simulink model "sim_env"  (R2023b)
settings: Solver=VariableStepAuto  StartTime=0.0  StopTime=10  RelTol=1e-3
values from neighbouring files (symbols this model uses):
  cg_z = 0.335    [para_sim1dot4.mat]    (also in para_sim1dot5.mat; para_sim1dot6.mat = 0.215; para_sim1dot7.mat = 0.215)
  F35thrust = [0 0.011 0.018 0.024 0.031 0.037 0.046 0.053 0.061 0.07 0.079 0.088 ... (170 elements, 85x2)]    [para_sim1dot3.mat]    (also in para_sim1dot4.mat; para_sim1dot5.mat; para_sim1dot6.mat; para_sim1dot7.mat)
  fin_drag_over_v2 = [-30 -25 -20 -15 -10 -5 0 5 10 15 20 25 ... (26 elements, 13x2)]    [para_sim1dot2.mat]    (also in para_sim1dot3.mat; para_sim1dot4.mat; para_sim1dot5.mat; para_sim1dot6.mat)
  fin_lift_over_v2 = [-30 -25 -20 -15 -10 -5 0 5 10 15 20 25 ... (26 elements, 13x2)]    [para_sim1dot2.mat]    (also in para_sim1dot3.mat; para_sim1dot4.mat; para_sim1dot5.mat; para_sim1dot6.mat)
  l_arm_moment = 0.5    [para_sim1dot2.mat]    (also in para_sim1dot3.mat; para_sim1dot4.mat = 0.3; para_sim1dot5.mat = 0.3; para_sim1dot6.mat = 0.175)
  mass = 1    [para_sim1dot0.mat]    (also in para_sim1dot1.mat; para_sim1dot2.mat = 0.6; para_sim1dot3.mat = 0.8; para_sim1dot4.mat = 0.8)
  r_arm_moment = 0.05    [para_sim1dot2.mat]    (also in para_sim1dot3.mat; para_sim1dot4.mat; para_sim1dot5.mat; para_sim1dot6.mat = 0.065)
libraries: simulink_extras x7, simulink x3, shared6dof x1, aerolibanim x1, matrix_library x1, aerolibanimutils x1
settings Model: Creator=Zian Liu  LastModifiedBy=Zian Liu

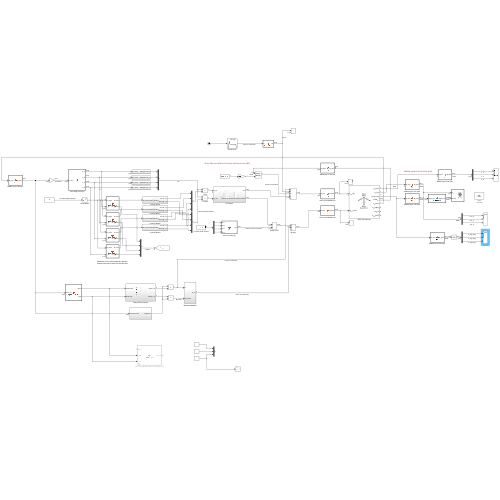
[thumbnail: Simulink's stored preview of the top-level diagram]
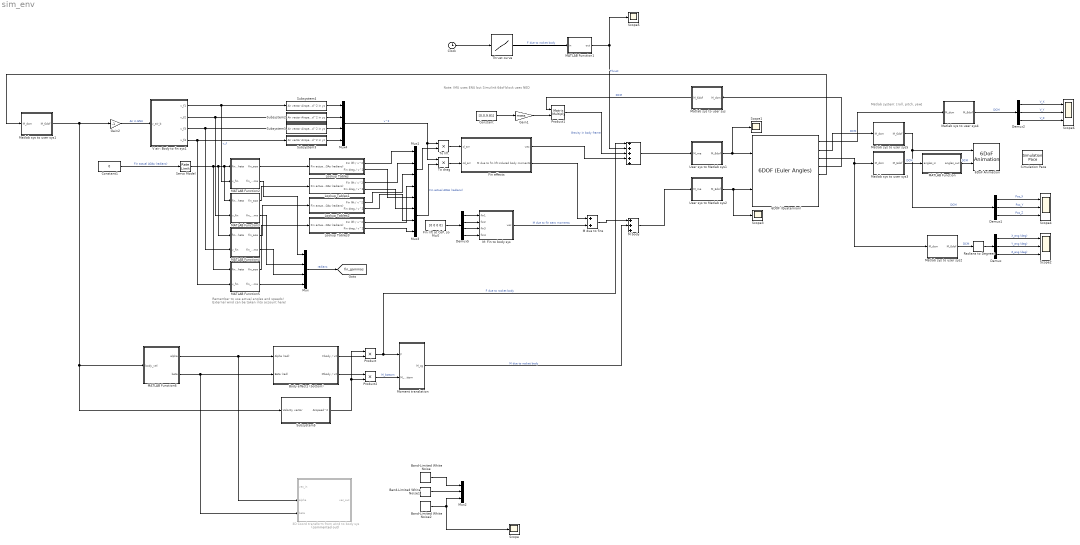
== system sim_env ==
  note: Matlab system: [roll, pitch, yaw]
  note: Note: IMU uses ENU but Simulink 6dof block uses NED
  note: Remember to use actual angles and speeds!
      | External wind can be taken into account here!
  " " : Sum  Inputs=+++++
  3D Coord transform from wind to body sys : MATLAB Function  Commented=on  TreatAsAtomicUnit=on
  6DOF (Quaternion) : shared6dof/6DOF (Euler Angles)  units=Metric (MKS)  mtype=Fixed  rep=Quaternion  xme_0=[0 0 0]  Vm_0=[0 0 0]  eul_0=[0 0 0]  pm_0=[0 0 0]  mass_0=mass  mass_e=0.5  mass_f=2.0  inertia=diag([0.0301315, 0.0301315, 0.0004096])  inertia_e=eye(3)  inertia_f=2*eye(3)  k_quat=1.0  vre_flag=on  abi_flag=off  aMode=0  xme_statename=''  Vm_statename=''  eul_statename=''  quat_statename={'qr', 'qi', 'qj','qk'}  pm_statename=''  mass_statename=''
      settings: LibrarySourceBlock=aerolib6dof2/6DOF (Quaternion)
  6DoF Animation : aerolibanim/6DoF Animation  u1=[-100 100 -100 100 -300 300]  u2=0.1  u3=100  u4=[10000 0 0]  u5=Fly alongside  u6=[10000 0 0]  u7=0  u8=off
  Band-Limited White Noise : simulink/Sources/Band-Limited White Noise  Cov=[0.1]  Ts=0.01  seed=[23341]
  Band-Limited White Noise1 : simulink/Sources/Band-Limited White Noise  Cov=[0.1]  Ts=0.01  seed=[23342]
  Band-Limited White Noise2 : simulink/Sources/Band-Limited White Noise  Cov=[0.1]  Ts=0.01  seed=[23343]
  Body effects (bottom) : Subsystem
  Clock : Clock
  Constant : Constant  Value=[0,0,9.81]
  Constant1 : Constant  Value=0
  Demux : Demux  Outputs=3
  Demux1 : Demux  Outputs=3
  Demux2 : Demux  Outputs=3
  Demux5 : Demux
  Fin effects : Subsystem
  "Fin lift at CoP, so M=0" : Constant  Value=[0 0 0 0]
  Gain1 : Gain  Gain=mass
  Gain2 : Gain  Gain=-1
  Lookup Tables : Subsystem
  Lookup Tables1 : Subsystem
  Lookup Tables2 : Subsystem
  Lookup Tables3 : Subsystem
  M body : Sum  Inputs=+++
  M due to fins : Sum
  M: Fin to body sys : MATLAB Function  TreatAsAtomicUnit=on
  MATLAB Function : MATLAB Function  TreatAsAtomicUnit=on
  MATLAB Function1 : MATLAB Function  TreatAsAtomicUnit=on
  MATLAB Function2 : MATLAB Function  TreatAsAtomicUnit=on
  MATLAB Function3 : MATLAB Function  TreatAsAtomicUnit=on
  MATLAB Function4 : MATLAB Function  TreatAsAtomicUnit=on
  MATLAB Function5 : MATLAB Function  TreatAsAtomicUnit=on
  MATLAB Function6 : MATLAB Function  TreatAsAtomicUnit=on
  Matlab sys to user sys : MATLAB Function  TreatAsAtomicUnit=on
  Matlab sys to user sys1 : MATLAB Function  TreatAsAtomicUnit=on
  Matlab sys to user sys2 : MATLAB Function  TreatAsAtomicUnit=on
  Matlab sys to user sys3 : MATLAB Function  TreatAsAtomicUnit=on
  Matlab sys to user sys4 : MATLAB Function  TreatAsAtomicUnit=on
  Matlab sys to user sys5 : MATLAB Function  TreatAsAtomicUnit=on
  Moment translation : Subsystem
  Mux{,1,3..4} (4 alike) : Mux
  Mux2 : Mux  Inputs=3
  Product : Product
  Product1 : Product  Multiplication=Matrix(*)
  Product2 : Product
  Radians to Degrees : simulink_extras/Transformations/Radians to Degrees
  Scope{,1,3,5} (4 alike) : Scope
  Scope2 : Scope  NumInputPorts=3
  Scope4 : Scope  NumInputPorts=3
  Scope6 : Scope  NumInputPorts=3
  Servo Model : RateLimiter  SampleTimeMode=inherited
  Simulation Pace : aerolibanimutils/Simulation Pace  SimulationPace=1  SleepMode=Auto  OutputPaceError=off  SampleTime=1/30
  Subsystem1 : Subsystem
  Subsystem2 : Subsystem
  Subsystem3 : Subsystem
  Subsystem4 : Subsystem
  Subsystem5 : Subsystem
  Thrust curve : Lookup_n-D  NumberOfTableDimensions=1  BreakpointsForDimension1=F35thrust(:,1)  Table=F35thrust(:,2)  ExtrapMethod=Clip  InternalRulePriority=Speed  RndMeth=Simplest
  To drag : Product
  To lift : Product
  User sys to Matlab sys1 : MATLAB Function  TreatAsAtomicUnit=on
  User sys to Matlab sys2 : MATLAB Function  TreatAsAtomicUnit=on
  V air: Body to fin sys1 : MATLAB Function  TreatAsAtomicUnit=on
  tag scope: fin_gammas=global
  wires:
  Matlab sys to user sys1/1(M_6dof) -> Subsystem5/1(Velocity vector), MATLAB Function6/1(body_vel), Gain2/1
  Gain2/1 -> V air: Body to fin sys1/1(v_air_b)  "Air in ENU"
  Subsystem1/1(Airspeed^2 in yz) -> Mux4/3
  Subsystem2/1(Airspeed^2 in yz) -> Mux4/2
  Mux1/1 -> To lift/2
  V air: Body to fin sys1/4(v_f4) -> Subsystem3/1(Air vector), MATLAB Function5/2(v_fin)
  Subsystem4/1(Airspeed^2 in yz) -> Mux4/1
  Matlab sys to user sys/1(M_6dof) -> Product1/1  "DCM"
  Constant1/1 -> Servo Model/1  "Fin actual AOAs (radians)"
  6DOF (Quaternion)/3 -> Matlab sys to user sys2/1(M_dcm), Matlab sys to user sys3/1(M_dcm)
  Subsystem3/1(Airspeed^2 in yz) -> Mux4/4
  Gain1/1 -> Product1/2
  M due to fins/1 -> M body/1
  " "/1 -> User sys to Matlab sys1/1(M_me)
  User sys to Matlab sys2/1(M_6dof) -> Scope3/1, 6DOF (Quaternion)/2
  Constant/1 -> Gain1/1
  "Fin lift at CoP, so M=0"/1 -> Demux5/1
  M body/1 -> User sys to Matlab sys2/1(M_me)
  V air: Body to fin sys1/3(v_f3) -> Subsystem1/1(Air vector), MATLAB Function4/2(v_fin)
  Moment translation/1(M_cg) -> M body/2  "M due to rocket body"
  Demux5/2 -> M: Fin to body sys/2(fin2)
  Demux5/3 -> M: Fin to body sys/3(fin3)
  Thrust curve/1 -> MATLAB Function1/1(in)  "F due to rocket body"
  Demux5/1 -> M: Fin to body sys/1(fin1)
  Demux5/4 -> M: Fin to body sys/4(fin4)
  M: Fin to body sys/1(vec) -> M due to fins/2  "M due to fin aero moments"
  User sys to Matlab sys1/1(M_6dof) -> 6DOF (Quaternion)/1, Scope1/1
  Mux4/1 -> To drag/1, To lift/1  "v^2"
  Product1/1 -> " "/3  "Gravity in body frame"
  6DOF (Quaternion)/4 -> Matlab sys to user sys/1(M_dcm)
  6DOF (Quaternion)/5 -> Matlab sys to user sys1/1(M_dcm)
  Matlab sys to user sys2/1(M_6dof) -> Radians to Degrees/1  "DCM"
  6DOF (Quaternion)/2 -> Matlab sys to user sys5/1(M_dcm)  "DCM"
  Clock/1 -> Thrust curve/1
  MATLAB Function1/1(out) -> Scope5/1, " "/2  "Thrust"
  MATLAB Function/1(angles_out) -> 6DoF Animation/2  "DCM"
  Matlab sys to user sys3/1(M_6dof) -> MATLAB Function/1(angles_in)  "DCM"
  Matlab sys to user sys5/1(M_6dof) -> Demux1/1, 6DoF Animation/1  "DCM"
  V air: Body to fin sys1/1(v_f1) -> Subsystem4/1(Air vector), MATLAB Function2/2(v_fin)  "v_f"
  V air: Body to fin sys1/2(v_f2) -> Subsystem2/1(Air vector), MATLAB Function3/2(v_fin)
  Demux/3 -> Scope2/3  "Z_ang (deg)"
  Demux/2 -> Scope2/2  "Y_ang (deg)"
  Demux/1 -> Scope2/1  "X_ang (deg)"
  Demux1/3 -> Scope4/3  "Pos_Z"
  Demux1/1 -> Scope4/1  "Pos_X"
  Demux1/2 -> Scope4/2  "Pos_Y"
  MATLAB Function2/1(fin_aoa) -> Lookup Tables/1(Fin actual AOAs (radians))
  MATLAB Function3/1(fin_aoa) -> Lookup Tables1/1(Fin actual AOAs (radians))
  MATLAB Function4/1(fin_aoa) -> Lookup Tables2/1(Fin actual AOAs (radians))
  MATLAB Function5/1(fin_aoa) -> Lookup Tables3/1(Fin actual AOAs (radians))
  MATLAB Function6/1(alpha) -> 3D Coord transform from wind to body sys/2(alpha), Body effects (bottom)/1(Alpha (rad))
  MATLAB Function6/2(beta) -> 3D Coord transform from wind to body sys/3(beta), Body effects (bottom)/2(Beta (rad))
  MATLAB Function5/2(fin_gamma) -> Mux/4
  To lift/1 -> Fin effects/1(cl_arr)
  To drag/1 -> Fin effects/2(cd_arr)
  Fin effects/1(vec) -> " "/4
  Fin effects/2(M due to fin lift induced body moments) -> M due to fins/1
  Mux/1 -> [fin_gammas]  "radians"
  MATLAB Function4/2(fin_gamma) -> Mux/3
  MATLAB Function3/2(fin_gamma) -> Mux/2
  MATLAB Function2/2(fin_gamma) -> Mux/1
  Band-Limited White Noise/1 -> Mux2/1
  Band-Limited White Noise2/1 -> Scope/1, Mux2/3
  Band-Limited White Noise1/1 -> Mux2/2
  Demux2/3 -> Scope6/3  "V_Z"
  Demux2/2 -> Scope6/2  "V_Y"
  Demux2/1 -> Scope6/1  "V_X"
  6DOF (Quaternion)/1 -> Matlab sys to user sys4/1(M_dcm)
  Matlab sys to user sys4/1(M_6dof) -> Demux2/1  "DCM"
  Servo Model/1 -> MATLAB Function5/1(fin_theta), MATLAB Function4/1(fin_theta), MATLAB Function3/1(fin_theta), MATLAB Function2/1(fin_theta)
  Lookup Tables/1(Fin lift / v^2) -> Mux1/1
  Lookup Tables1/1(Fin lift / v^2) -> Mux1/2
  Lookup Tables2/1(Fin lift / v^2) -> Mux1/3
  Lookup Tables3/1(Fin lift / v^2) -> Mux1/4
  Lookup Tables/2(Fin drag / v^2) -> Mux3/1
  Lookup Tables1/2(Fin drag / v^2) -> Mux3/2
  Lookup Tables2/2(Fin drag / v^2) -> Mux3/3
  Lookup Tables3/2(Fin drag / v^2) -> Mux3/4
  Mux3/1 -> To drag/2  "Fin actual AOAs (radians)"
  Radians to Degrees/1 -> Demux/1
  Product2/1 -> Moment translation/2(M_bottom)  "M_bottom"
  Product/1 -> Moment translation/1(F), " "/1  "F due to rocket body"
  Body effects (bottom)/1(Fbody / v2) -> Product/2
  Body effects (bottom)/2(Mbody / v2) -> Product2/1
  Subsystem5/1(Airspeed^2) -> Product/1, Product2/2

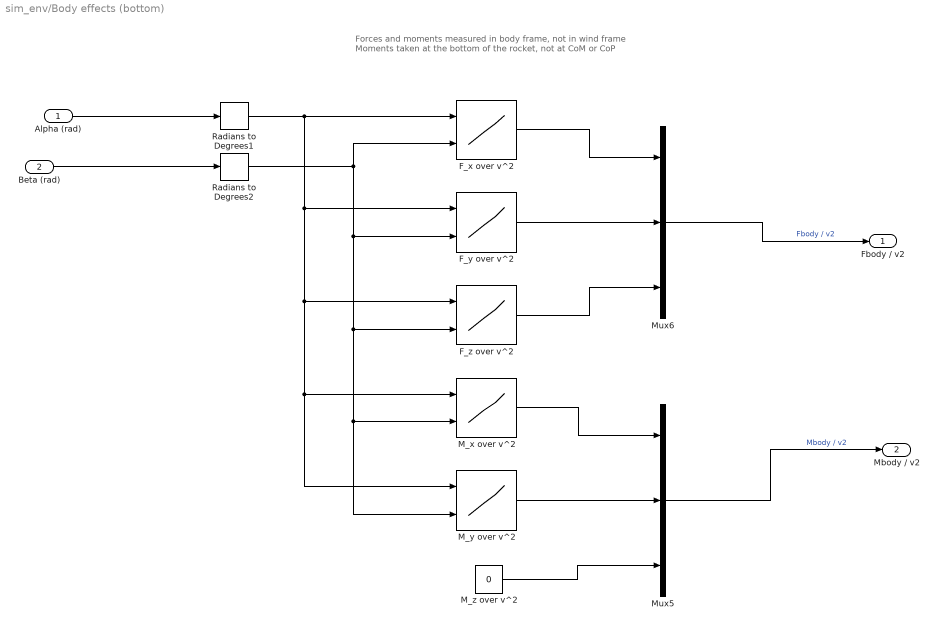
== system sim_env/Body effects (bottom) ==
  note: Forces and moments measured in body frame, not in wind frame
      |
      | Moments taken at the bottom of the rocket, not at CoM or CoP
  Alpha (rad) : Inport
  Beta (rad) : Inport  Port=2
  F_x over v^2 : Lookup_n-D  BreakpointsForDimension1=body_Fx_over_v2(2:end,1)  BreakpointsForDimension2=body_Fx_over_v2(1,2:end)  BreakpointsForDimension3=[5, 7]  Table=body_Fx_over_v2(2:end,2:end)  ExtrapMethod=Clip  InternalRulePriority=Speed  RndMeth=Simplest
      settings: InputPortMap=u0,u1
  F_y over v^2 : Lookup_n-D  BreakpointsForDimension1=body_Fy_over_v2(2:end,1)  BreakpointsForDimension2=body_Fy_over_v2(1,2:end)  BreakpointsForDimension3=[5, 7]  Table=body_Fy_over_v2(2:end,2:end)  ExtrapMethod=Clip  InternalRulePriority=Speed  RndMeth=Simplest
      settings: InputPortMap=u0,u1
  F_z over v^2 : Lookup_n-D  BreakpointsForDimension1=body_Fz_over_v2(2:end,1)  BreakpointsForDimension2=body_Fz_over_v2(1,2:end)  BreakpointsForDimension3=[5, 7]  Table=body_Fz_over_v2(2:end,2:end)  ExtrapMethod=Clip  InternalRulePriority=Speed  RndMeth=Simplest
      settings: InputPortMap=u0,u1
  M_x over v^2 : Lookup_n-D  BreakpointsForDimension1=body_Mx_over_v2(2:end,1)  BreakpointsForDimension2=body_Mx_over_v2(1,2:end)  BreakpointsForDimension3=[5, 7]  Table=body_Mx_over_v2(2:end,2:end)  ExtrapMethod=Clip  InternalRulePriority=Speed  RndMeth=Simplest
      settings: InputPortMap=u0,u1
  M_y over v^2 : Lookup_n-D  BreakpointsForDimension1=body_My_over_v2(2:end,1)  BreakpointsForDimension2=body_My_over_v2(1,2:end)  BreakpointsForDimension3=[5, 7]  Table=body_My_over_v2(2:end,2:end)  ExtrapMethod=Clip  InternalRulePriority=Speed  RndMeth=Simplest
      settings: InputPortMap=u0,u1
  M_z over v^2 : Constant  Value=0
  Mux5 : Mux  Inputs=3
  Mux6 : Mux  Inputs=3
  Radians to Degrees1 : simulink_extras/Transformations/Radians to Degrees
  Radians to Degrees2 : simulink_extras/Transformations/Radians to Degrees
  Fbody / v2 : Outport
  Mbody / v2 : Outport  Port=2
  wires:
  F_y over v^2/1 -> Mux6/2
  M_x over v^2/1 -> Mux5/1
  Radians to Degrees1/1 -> M_y over v^2/1, M_x over v^2/1, F_z over v^2/1, F_y over v^2/1, F_x over v^2/1
  Radians to Degrees2/1 -> F_x over v^2/2, M_y over v^2/2, M_x over v^2/2, F_z over v^2/2, F_y over v^2/2
  F_x over v^2/1 -> Mux6/1
  Mux6/1 -> Fbody / v2/1  "Fbody / v2"
  M_y over v^2/1 -> Mux5/2
  Alpha (rad)/1 -> Radians to Degrees1/1
  M_z over v^2/1 -> Mux5/3
  F_z over v^2/1 -> Mux6/3
  Mux5/1 -> Mbody / v2/1  "Mbody / v2"
  Beta (rad)/1 -> Radians to Degrees2/1

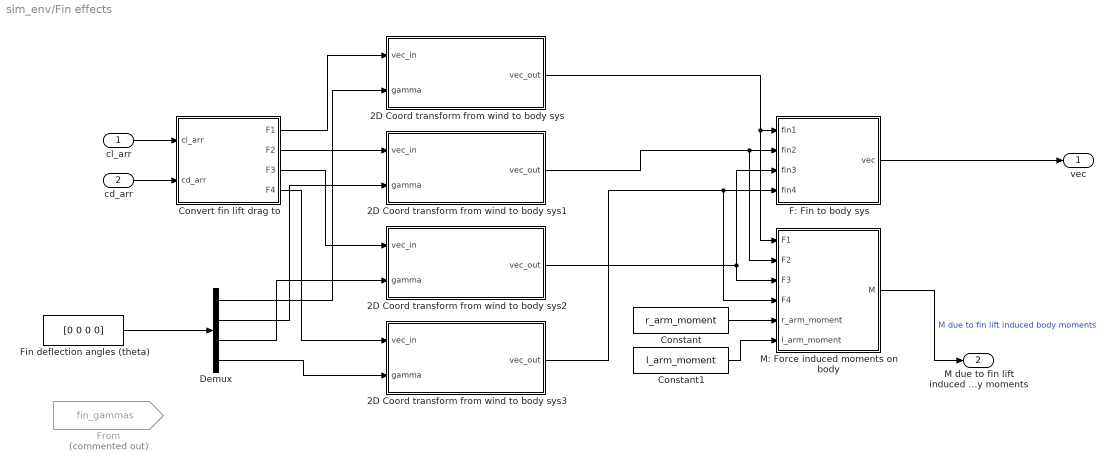
== system sim_env/Fin effects ==
  cl_arr : Inport
  cd_arr : Inport  Port=2
  2D Coord transform from wind to body sys : MATLAB Function  TreatAsAtomicUnit=on
  2D Coord transform from wind to body sys1 : MATLAB Function  TreatAsAtomicUnit=on
  2D Coord transform from wind to body sys2 : MATLAB Function  TreatAsAtomicUnit=on
  2D Coord transform from wind to body sys3 : MATLAB Function  TreatAsAtomicUnit=on
  Constant : Constant  Value=r_arm_moment
  Constant1 : Constant  Value=l_arm_moment
  "Convert fin lift drag to " : MATLAB Function  TreatAsAtomicUnit=on
  Demux : Demux
  F: Fin to body sys : MATLAB Function  TreatAsAtomicUnit=on
  Fin deflection angles (theta) : Constant  Value=[0 0 0 0]
  From : From  Commented=on  GotoTag=fin_gammas  TagVisibility=global
  M: Force induced moments on body : MATLAB Function  TreatAsAtomicUnit=on
  vec : Outport
  M due to fin lift induced body moments : Outport  Port=2
  wires:
  2D Coord transform from wind to body sys/1(vec_out) -> M: Force induced moments on body/1(F1), F: Fin to body sys/1(fin1)
  2D Coord transform from wind to body sys2/1(vec_out) -> F: Fin to body sys/3(fin3), M: Force induced moments on body/3(F3)
  2D Coord transform from wind to body sys3/1(vec_out) -> M: Force induced moments on body/4(F4), F: Fin to body sys/4(fin4)
  cl_arr/1 -> "Convert fin lift drag to "/1(cl_arr)
  2D Coord transform from wind to body sys1/1(vec_out) -> M: Force induced moments on body/2(F2), F: Fin to body sys/2(fin2)
  F: Fin to body sys/1(vec) -> vec/1
  M: Force induced moments on body/1(M) -> M due to fin lift induced body moments/1  "M due to fin lift induced body moments"
  cd_arr/1 -> "Convert fin lift drag to "/2(cd_arr)
  "Convert fin lift drag to "/1(F1) -> 2D Coord transform from wind to body sys/1(vec_in)
  "Convert fin lift drag to "/2(F2) -> 2D Coord transform from wind to body sys1/1(vec_in)
  "Convert fin lift drag to "/3(F3) -> 2D Coord transform from wind to body sys2/1(vec_in)
  "Convert fin lift drag to "/4(F4) -> 2D Coord transform from wind to body sys3/1(vec_in)
  Fin deflection angles (theta)/1 -> Demux/1
  Demux/4 -> 2D Coord transform from wind to body sys3/2(gamma)
  Demux/3 -> 2D Coord transform from wind to body sys2/2(gamma)
  Demux/2 -> 2D Coord transform from wind to body sys1/2(gamma)
  Demux/1 -> 2D Coord transform from wind to body sys/2(gamma)
  Constant/1 -> M: Force induced moments on body/5(r_arm_moment)
  Constant1/1 -> M: Force induced moments on body/6(l_arm_moment)

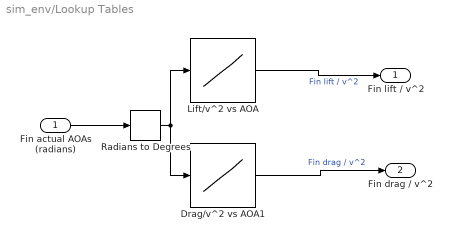
== system sim_env/Lookup Tables ==
  Fin actual AOAs (radians) : Inport
  Drag/v^2 vs AOA1 : Lookup_n-D  NumberOfTableDimensions=1  BreakpointsForDimension1=fin_drag_over_v2(:,1)  Table=fin_drag_over_v2(:,2)  ExtrapMethod=Clip  InternalRulePriority=Speed  RndMeth=Simplest
  Lift/v^2 vs AOA : Lookup_n-D  NumberOfTableDimensions=1  BreakpointsForDimension1=fin_lift_over_v2(:,1)  Table=fin_lift_over_v2(:,2)  ExtrapMethod=Clip  InternalRulePriority=Speed  RndMeth=Simplest
  Radians to Degrees : simulink_extras/Transformations/Radians to Degrees
  Fin lift / v^2 : Outport
  Fin drag / v^2 : Outport  Port=2
  wires:
  Radians to Degrees/1 -> Lift/v^2 vs AOA/1, Drag/v^2 vs AOA1/1
  Drag/v^2 vs AOA1/1 -> Fin drag / v^2/1  "Fin drag / v^2"
  Lift/v^2 vs AOA/1 -> Fin lift / v^2/1  "Fin lift / v^2"
  Fin actual AOAs (radians)/1 -> Radians to Degrees/1

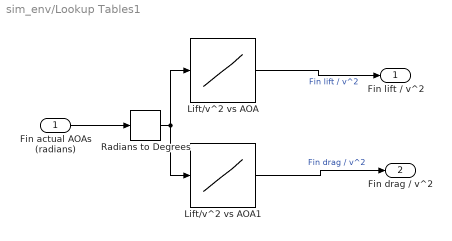
== system sim_env/Lookup Tables1 ==
  Fin actual AOAs (radians) : Inport
  Lift/v^2 vs AOA : Lookup_n-D  NumberOfTableDimensions=1  BreakpointsForDimension1=fin_lift_over_v2(:,1)  Table=fin_lift_over_v2(:,2)  ExtrapMethod=Clip  InternalRulePriority=Speed  RndMeth=Simplest
  Lift/v^2 vs AOA1 : Lookup_n-D  NumberOfTableDimensions=1  BreakpointsForDimension1=fin_drag_over_v2(:,1)  Table=fin_drag_over_v2(:,2)  ExtrapMethod=Clip  InternalRulePriority=Speed  RndMeth=Simplest
  Radians to Degrees : simulink_extras/Transformations/Radians to Degrees
  Fin lift / v^2 : Outport
  Fin drag / v^2 : Outport  Port=2
  wires:
  Radians to Degrees/1 -> Lift/v^2 vs AOA/1, Lift/v^2 vs AOA1/1
  Lift/v^2 vs AOA1/1 -> Fin drag / v^2/1  "Fin drag / v^2"
  Lift/v^2 vs AOA/1 -> Fin lift / v^2/1  "Fin lift / v^2"
  Fin actual AOAs (radians)/1 -> Radians to Degrees/1

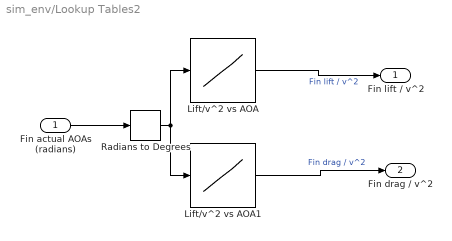
== system sim_env/Lookup Tables2 ==
  Fin actual AOAs (radians) : Inport
  Lift/v^2 vs AOA : Lookup_n-D  NumberOfTableDimensions=1  BreakpointsForDimension1=fin_lift_over_v2(:,1)  Table=fin_lift_over_v2(:,2)  ExtrapMethod=Clip  InternalRulePriority=Speed  RndMeth=Simplest
  Lift/v^2 vs AOA1 : Lookup_n-D  NumberOfTableDimensions=1  BreakpointsForDimension1=fin_drag_over_v2(:,1)  Table=fin_drag_over_v2(:,2)  ExtrapMethod=Clip  InternalRulePriority=Speed  RndMeth=Simplest
  Radians to Degrees : simulink_extras/Transformations/Radians to Degrees
  Fin lift / v^2 : Outport
  Fin drag / v^2 : Outport  Port=2
  wires:
  Radians to Degrees/1 -> Lift/v^2 vs AOA/1, Lift/v^2 vs AOA1/1
  Lift/v^2 vs AOA1/1 -> Fin drag / v^2/1  "Fin drag / v^2"
  Lift/v^2 vs AOA/1 -> Fin lift / v^2/1  "Fin lift / v^2"
  Fin actual AOAs (radians)/1 -> Radians to Degrees/1

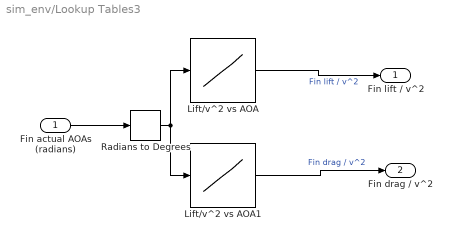
== system sim_env/Lookup Tables3 ==
  Fin actual AOAs (radians) : Inport
  Lift/v^2 vs AOA : Lookup_n-D  NumberOfTableDimensions=1  BreakpointsForDimension1=fin_lift_over_v2(:,1)  Table=fin_lift_over_v2(:,2)  ExtrapMethod=Clip  InternalRulePriority=Speed  RndMeth=Simplest
  Lift/v^2 vs AOA1 : Lookup_n-D  NumberOfTableDimensions=1  BreakpointsForDimension1=fin_drag_over_v2(:,1)  Table=fin_drag_over_v2(:,2)  ExtrapMethod=Clip  InternalRulePriority=Speed  RndMeth=Simplest
  Radians to Degrees : simulink_extras/Transformations/Radians to Degrees
  Fin lift / v^2 : Outport
  Fin drag / v^2 : Outport  Port=2
  wires:
  Radians to Degrees/1 -> Lift/v^2 vs AOA/1, Lift/v^2 vs AOA1/1
  Lift/v^2 vs AOA1/1 -> Fin drag / v^2/1  "Fin drag / v^2"
  Lift/v^2 vs AOA/1 -> Fin lift / v^2/1  "Fin lift / v^2"
  Fin actual AOAs (radians)/1 -> Radians to Degrees/1

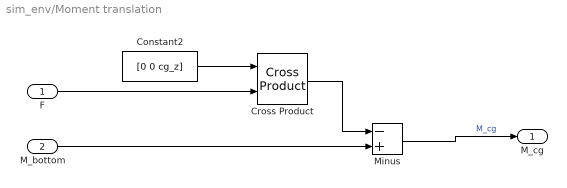
== system sim_env/Moment translation ==
  F : Inport
  M_bottom : Inport  Port=2
  Constant2 : Constant  Value=[0 0 cg_z]
  Cross Product : matrix_library/Cross Product
  Minus : Sum  Inputs=-+
  M_cg : Outport
  wires:
  F/1 -> Cross Product/2
  Cross Product/1 -> Minus/1
  Constant2/1 -> Cross Product/1
  Minus/1 -> M_cg/1  "M_cg"
  M_bottom/1 -> Minus/2

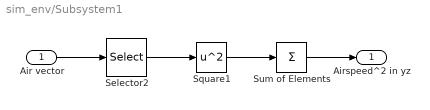
== system sim_env/Subsystem1 ==
  Air vector : Inport
  Selector2 : Selector  InputPortWidth=3  IndexOptions=Index vector (dialog)  Indices=[2 3]  OutputSizes=1
  Square1 : Math  Operator=square
  Sum of Elements : Sum  Inputs=+
  Airspeed^2 in yz : Outport
  wires:
  Square1/1 -> Sum of Elements/1
  Selector2/1 -> Square1/1
  Sum of Elements/1 -> Airspeed^2 in yz/1
  Air vector/1 -> Selector2/1

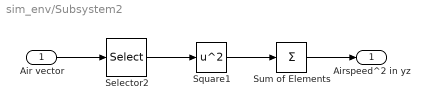
== system sim_env/Subsystem2 ==
  Air vector : Inport
  Selector2 : Selector  InputPortWidth=3  IndexOptions=Index vector (dialog)  Indices=[2 3]  OutputSizes=1
  Square1 : Math  Operator=square
  Sum of Elements : Sum  Inputs=+
  Airspeed^2 in yz : Outport
  wires:
  Square1/1 -> Sum of Elements/1
  Selector2/1 -> Square1/1
  Sum of Elements/1 -> Airspeed^2 in yz/1
  Air vector/1 -> Selector2/1

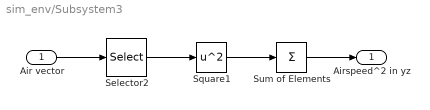
== system sim_env/Subsystem3 ==
  Air vector : Inport
  Selector2 : Selector  InputPortWidth=3  IndexOptions=Index vector (dialog)  Indices=[2 3]  OutputSizes=1
  Square1 : Math  Operator=square
  Sum of Elements : Sum  Inputs=+
  Airspeed^2 in yz : Outport
  wires:
  Square1/1 -> Sum of Elements/1
  Selector2/1 -> Square1/1
  Sum of Elements/1 -> Airspeed^2 in yz/1
  Air vector/1 -> Selector2/1

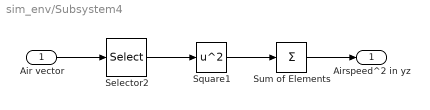
== system sim_env/Subsystem4 ==
  Air vector : Inport
  Selector2 : Selector  InputPortWidth=3  IndexOptions=Index vector (dialog)  Indices=[2 3]  OutputSizes=1
  Square1 : Math  Operator=square
  Sum of Elements : Sum  Inputs=+
  Airspeed^2 in yz : Outport
  wires:
  Square1/1 -> Sum of Elements/1
  Selector2/1 -> Square1/1
  Sum of Elements/1 -> Airspeed^2 in yz/1
  Air vector/1 -> Selector2/1

== system sim_env/Subsystem5 ==
  Velocity vector : Inport
  Square1 : Math  Operator=square
  Sum of Elements : Sum  Inputs=+
  Airspeed^2 : Outport
  wires:
  Square1/1 -> Sum of Elements/1
  Velocity vector/1 -> Square1/1
  Sum of Elements/1 -> Airspeed^2/1

== matlab function sim_env/MATLAB Function ==
  data: angles_in input; angles_out output
function angles_out = pitchadd2pi(angles_in)
angles_out = [angles_in(1); angles_in(2)-pi/2; angles_in(3)];

== matlab function sim_env/MATLAB Function1 ==
  data: in input; out output
function out = thrustz2vec(in)
out = [0 0 in];

== matlab function sim_env/Matlab sys to user sys3 ==
  data: M_dcm input; M_6dof output
function M_6dof = fcn(M_dcm)
M_lab2user = [0 1 0; 1 0 0; 0 0 -1];
M_6dof = M_lab2user * M_dcm;

== matlab function sim_env/MATLAB Function2 ==
  data: fin_theta input; fin_aoa output; v_fin input; fin_gamma output
function [fin_aoa, fin_gamma]= theta2aoa_fin(fin_theta, v_fin)
vz = v_fin(3);
vy = v_fin(2);
fin_gamma = - pi/2 - atan2(vz, vy); % assuming v_fin points in q3 or q4 (negative z) during launch, note vz cannot points upwards, or gamma will be big in q2
fin_aoa = fin_theta - fin_gamma;

== matlab function sim_env/Matlab sys to user sys5 ==
  data: M_dcm input; M_6dof output
function M_6dof = fcn(M_dcm)
M_lab2user = [0 1 0; 1 0 0; 0 0 -1];
M_6dof = M_lab2user * M_dcm;

== matlab function sim_env/MATLAB Function3 ==
  data: fin_theta input; fin_aoa output; v_fin input; fin_gamma output
function [fin_aoa, fin_gamma]= theta2aoa_fin(fin_theta, v_fin)
vz = v_fin(3);
vy = v_fin(2);
fin_gamma = - pi/2 - atan2(vz, vy); % assuming v_fin points in q3 or q4 (negative z) during launch, note vz cannot points upwards, or gamma will be big in q2
fin_aoa = fin_theta - fin_gamma;

== matlab function sim_env/MATLAB Function4 ==
  data: fin_theta input; fin_aoa output; v_fin input; fin_gamma output
function [fin_aoa, fin_gamma]= theta2aoa_fin(fin_theta, v_fin)
vz = v_fin(3);
vy = v_fin(2);
fin_gamma = - pi/2 - atan2(vz, vy); % assuming v_fin points in q3 or q4 (negative z) during launch, note vz cannot points upwards, or gamma will be big in q2
fin_aoa = fin_theta - fin_gamma;

== matlab function sim_env/MATLAB Function5 ==
  data: fin_theta input; fin_aoa output; v_fin input; fin_gamma output
function [fin_aoa, fin_gamma]= theta2aoa_fin(fin_theta, v_fin)
vz = v_fin(3);
vy = v_fin(2);
fin_gamma = - pi/2 - atan2(vz, vy); % assuming v_fin points in q3 or q4 (negative z) during launch, note vz cannot points upwards, or gamma will be big in q2
fin_aoa = fin_theta - fin_gamma;

== matlab function sim_env/Fin effects/F: Fin to body sys ==
  data: fin1 input; vec output; fin2 input; fin3 input; fin4 input
function vec = fcn(fin1, fin2, fin3, fin4)
vx = fin1(1) - fin2(2) - fin3(1) + fin4(2);
vy = fin1(2) + fin2(1) - fin3(2) - fin4(1);
vz = fin1(3) + fin2(3) + fin3(3) + fin4(3);

vec = [vx, vy, vz];

== matlab function sim_env/MATLAB Function6 ==
  data: body_vel input; alpha output; beta output
function [alpha, beta]= alpha_beta_rad(body_vel)
vt = norm(body_vel);
vx = body_vel(1);
vy = body_vel(2);
beta = asin(vx / vt);
alpha = asin(vy / (vt * cos(beta)));

== matlab function sim_env/3D Coord transform from wind to body sys ==
  data: vec_in input; vec_out output; alpha input; beta input
function vec_out = wind2body(vec_in, alpha, beta)
vec_in_T = transpose(vec_in);
vec_out = [cos(alpha), 0, -sin(alpha);
           0,          1,  0;
           sin(alpha), 0,  cos(alpha)] * ...
          [cos(beta), -sin(beta), 0;
          sin(beta),  cos(beta), 0;
          0,          0,         1] * vec_in_T;

== matlab function sim_env/Fin effects/2D Coord transform from wind to body sys ==
  data: vec_in input; vec_out output; gamma input
function vec_out = wind2body_fin(vec_in, gamma) % beta converts vec in wind sys to 0 fin angle sys which is parallel to rocket body sys

vec_in_T = transpose(vec_in);
vec_out = [1, 0,         0;
           0, cos(gamma), -sin(gamma);
           0, sin(gamma), cos(gamma),] * vec_in_T;

== matlab function sim_env/Fin effects/2D Coord transform from wind to body sys1 ==
  data: vec_in input; vec_out output; gamma input
function vec_out = wind2body_fin(vec_in, gamma) % beta converts vec in wind sys to 0 fin angle sys which is parallel to rocket body sys

vec_in_T = transpose(vec_in);
vec_out = [1, 0,         0;
           0, cos(gamma), -sin(gamma);
           0, sin(gamma), cos(gamma),] * vec_in_T;

== matlab function sim_env/Fin effects/2D Coord transform from wind to body sys2 ==
  data: vec_in input; vec_out output; gamma input
function vec_out = wind2body_fin(vec_in, gamma) % beta converts vec in wind sys to 0 fin angle sys which is parallel to rocket body sys

vec_in_T = transpose(vec_in);
vec_out = [1, 0,         0;
           0, cos(gamma), -sin(gamma);
           0, sin(gamma), cos(gamma),] * vec_in_T;

== matlab function sim_env/Fin effects/2D Coord transform from wind to body sys3 ==
  data: vec_in input; vec_out output; gamma input
function vec_out = wind2body_fin(vec_in, gamma) % beta converts vec in wind sys to 0 fin angle sys which is parallel to rocket body sys

vec_in_T = transpose(vec_in);
vec_out = [1, 0,         0;
           0, cos(gamma), -sin(gamma);
           0, sin(gamma), cos(gamma),] * vec_in_T;

== matlab function sim_env/Matlab sys to user sys4 ==
  data: M_dcm input; M_6dof output
function M_6dof = fcn(M_dcm)
M_lab2user = [0 1 0; 1 0 0; 0 0 -1];
M_6dof = M_lab2user * M_dcm;

== matlab function sim_env/Matlab sys to user sys1 ==
  data: M_dcm input; M_6dof output
function M_6dof = fcn(M_dcm)
M_lab2user = [0 1 0; 1 0 0; 0 0 -1];
M_6dof = M_lab2user * M_dcm;

== matlab function sim_env/M: Fin to body sys ==
  data: fin1 input; vec output; fin2 input; fin3 input; fin4 input
function vec = fcn(fin1, fin2, fin3, fin4)
vx = -fin1 + fin3; % CW moment is positive, in negative x dir
vy = -fin2 + fin4;
vz = 0;

vec = [vx, vy, vz];

== matlab function sim_env/Fin effects/M: Force induced moments on body ==
  data: F1 input; M output; F2 input; F3 input; F4 input; r_arm_moment input; l_arm_moment input
function M = fcn(F1, F2, F3, F4, r_arm_moment, l_arm_moment)

r1 = [r_arm_moment, 0, -l_arm_moment];
r2 = [0, r_arm_moment, -l_arm_moment];
r3 = [-r_arm_moment, 0, -l_arm_moment];
r4 = [0, -r_arm_moment, -l_arm_moment];

F1_body = F1;
F2_body = [-F2(2) F2(1) F2(3)];
F3_body = [-F3(1) -F3(2) F3(3)];
F4_body = [F4(2) -F4(1) F4(3)];
M = cross(r1, F1_body) + cross(r2, F2_body) + cross(r3, F3_body) + cross(r4, F4_body);

== matlab function sim_env/Fin effects/Convert fin lift drag to  ==
  data: cl_arr input; F1 output; cd_arr input; F2 output; F3 output; F4 output
function [F1, F2, F3, F4]= fcn(cl_arr, cd_arr)
F1 = [0, cl_arr(1), -cd_arr(1)];
F2 = [0, cl_arr(2), -cd_arr(2)];
F3 = [0, cl_arr(3), -cd_arr(3)];
F4 = [0, cl_arr(4), -cd_arr(4)];

== matlab function sim_env/User sys to Matlab sys2 ==
  data: M_me input; M_6dof output
function M_6dof = fcn(M_me)
M_6dof = [M_me(2), M_me(1), -M_me(3)];

== matlab function sim_env/User sys to Matlab sys1 ==
  data: M_me input; M_6dof output
function M_6dof = fcn(M_me)
M_6dof = [M_me(2), M_me(1), -M_me(3)];

== matlab function sim_env/V air: Body to fin sys1 ==
  data: v_air_b input; v_f1 output; v_f2 output; v_f3 output; v_f4 output
function [v_f1, v_f2, v_f3, v_f4]= fcn(v_air_b)
vx = v_air_b(1);
vy = v_air_b(2);
vz = v_air_b(3);

v_f1 = [vx, vy, vz];
v_f2 = [vy, -vx, vz];
v_f3 = [-vx, -vy, vz];
v_f4 = [-vy, vx, vz];

== matlab function sim_env/Matlab sys to user sys ==
  data: M_dcm input; M_6dof output
function M_6dof = fcn(M_dcm)
M_lab2user = [0 1 0; 1 0 0; 0 0 -1];
M_6dof = M_lab2user * M_dcm;

== matlab function sim_env/Matlab sys to user sys2 ==
  data: M_dcm input; M_6dof output
function M_6dof = fcn(M_dcm)
M_lab2user = [0 1 0; 1 0 0; 0 0 -1];
M_6dof = M_lab2user * M_dcm;
